simulink model "ModeAdjust"  (R2018b)
settings: Solver=FixedStepDiscrete  StartTime=0.0  StopTime=inf  FixedStep=0.01  RelTol=1e-3
undefined symbols (not defined in the file or in its folder): IfKeSMSbSeatMovBkRclnEnable_Val, IfKeSMSbSeatMovFrwdBkwdEnable_Val, IfKeSMSbSeatMovFtrstEnable_Val, IfKeSMSbSeatMovHdrstFrwdBkwdEnable_Val, IfKeSMSbSeatMovHdUpwdDnwdEnable_Val, IfKeSMSbSeatMovLgrstEnable_Val, IfKeSMSbSeatMovLtwdRtwdEnable_Val, IfVeSMSeStNumConfig, KeSMSbArmscreenMovEnable_Val, KeSMSbSeatMovLgrstExpdEnable_Val, KeSMSuFirstRwStBackPosDelta_Val, KeSMSuFirstRwStBackPosTolr_Val, KeSMSuFirstRwStCushFrntPosDelta_Val, KeSMSuFirstRwStCushFrntPosTolr_Val, KeSMSuFirstRwStCushRePosDelta_Val, KeSMSuFirstRwStCushRePosTolr_Val, KeSMSuFirstRwStFootrestPosDelta_Val, KeSMSuFirstRwStFootrestPosTolr_Val, KeSMSuFirstRwStFwdBkwdPosDelta_Val, KeSMSuFirstRwStFwdBkwdPosTolr_Val, KeSMSuMdMotFinshdTm_Val, KeSMSuMdRetryTm1_Val, KeSMSuModeReqDurgTm_Val, KeSMSuSecRwStArmTochPosDelta_Val, KeSMSuSecRwStArmTochPosTolr_Val, KeSMSuSecRwStBackPosDelta_Val, KeSMSuSecRwStBackPosTolr_Val, KeSMSuSecRwStFtrstUpwdDnwdPosDelta_Val, KeSMSuSecRwStFtrstUpwdDnwdPosTolr_Val, KeSMSuSecRwStFwdBkwdPosDelta_Val, KeSMSuSecRwStFwdBkwdPosTolr_Val, KeSMSuSecRwStHeadrestFwdBkwdPosDelta_Val, KeSMSuSecRwStHeadrestFwdBkwdPosTolr_Val, KeSMSuSecRwStHeadrestUpwdDwnwdPosDelta_Val, KeSMSuSecRwStHeadrestUpwdDwnwdPosTolr_Val, KeSMSuSecRwStLegrestInOutPosDelta_Val, KeSMSuSecRwStLegrestInOutPosTolr_Val, KeSMSuSecRwStLegrestUpwdDwnwdPosDelta_Val, KeSMSuSecRwStLegrestUpwdDwnwdPosTolr_Val, KeSMSuSecRwStLwdRwdPosDelta_Val, KeSMSuSecRwStLwdRwdPosTolr_Val, KeSMSuSecRwStVIPFtrstRefAngle_Val, KeSMSuThirdRwStFwdBkwdPosDelta_Val, KeSMSuThirdRwStFwdBkwdPosTolr_Val, KeSMSuThrdRwCushFoldPosDelta_Val, KeSMSuThrdRwCushFoldPosTolr_Val, KeSMSuThrdRwStBackPosDelta_Val, KeSMSuThrdRwStBackPosTolr_Val, KeSMSw4SLegrstCloseMdSecRwLtStFtrstUpwdDnwdPos_Val, KeSMSw4SLegrstCloseMdSecRwLtStFtrstUpwdDnwdPosMax_Val, KeSMSw4SLegrstCloseMdSecRwLtStFtrstUpwdDnwdPosMin_Val, KeSMSw4SLegrstCloseMdSecRwLtStLgrstOtwdInwdPos_Val, KeSMSw4SLegrstCloseMdSecRwLtStLgrstOtwdInwdPosMax_Val, KeSMSw4SLegrstCloseMdSecRwLtStLgrstOtwdInwdPosMin_Val, KeSMSw4SLegrstCloseMdSecRwLtStLgrstUpwdDnwdPos_Val, KeSMSw4SLegrstCloseMdSecRwLtStLgrstUpwdDnwdPosMax_Val, KeSMSw4SLegrstCloseMdSecRwLtStLgrstUpwdDnwdPosMin_Val, KeSMSw4SLegrstCloseMdSecRwRtStFtrstUpwdDnwdPos_Val, KeSMSw4SLegrstCloseMdSecRwRtStFtrstUpwdDnwdPosMax_Val, KeSMSw4SLegrstCloseMdSecRwRtStFtrstUpwdDnwdPosMin_Val ... (+1138)
libraries: Lib x401
(part 7 of 35)

== system ModeAdjust/ModeAdjustRunnable_sys/ModeAdjust/Default ==
  Bus Creator : BusCreator  Inputs=36  OutDataTypeStr=Bus: isAcsMdFeedBack_Default
  Constant{,43..45} (4 alike) : Constant  Value=0  OutDataTypeStr=uint8
  Constant{1..42} (42 alike) : Constant  Value=0  OutDataTypeStr=boolean
  PA_KeSMSuFirstRwStBackPosDelta_Val : Constant  Value=KeSMSuFirstRwStBackPosDelta_Val
  PA_KeSMSuFirstRwStCushFrntPosDelta_Val : Constant  Value=KeSMSuFirstRwStCushFrntPosDelta_Val
  PA_KeSMSuFirstRwStCushRePosDelta_Val : Constant  Value=KeSMSuFirstRwStCushRePosDelta_Val
  PA_KeSMSuFirstRwStFootrestPosDelta_Val : Constant  Value=KeSMSuFirstRwStFootrestPosDelta_Val
  PA_KeSMSuFirstRwStFwdBkwdPosDelta_Val : Constant  Value=KeSMSuFirstRwStFwdBkwdPosDelta_Val
  PA_KeSMSuMdMotFinshdTm_Val : Constant  Value=KeSMSuMdMotFinshdTm_Val
  PA_KeSMSuSecRwStArmTochPosDelta_Val : Constant  Value=KeSMSuSecRwStArmTochPosDelta_Val
  PA_KeSMSuSecRwStBackPosDelta_Val : Constant  Value=KeSMSuSecRwStBackPosDelta_Val
  PA_KeSMSuSecRwStFwdBkwdPosDelta_Val : Constant  Value=KeSMSuSecRwStFwdBkwdPosDelta_Val
  PA_KeSMSuSecRwStHeadrestFwdBkwdPosDelta_Val : Constant  Value=KeSMSuSecRwStHeadrestFwdBkwdPosDelta_Val
  PA_KeSMSuSecRwStHeadrestUpwdDwnwdPosDelta_Val : Constant  Value=KeSMSuSecRwStHeadrestUpwdDwnwdPosDelta_Val
  PA_KeSMSuSecRwStLegrestInOutPosDelta_Val : Constant  Value=KeSMSuSecRwStLegrestInOutPosDelta_Val
  PA_KeSMSuSecRwStLegrestUpwdDwnwdPosDelta_Val : Constant  Value=KeSMSuSecRwStLegrestUpwdDwnwdPosDelta_Val
  PA_KeSMSuSecRwStLwdRwdPosDelta_Val : Constant  Value=KeSMSuSecRwStLwdRwdPosDelta_Val
  PA_KeSMSuThirdRwStFwdBkwdPosDelta_Val : Constant  Value=KeSMSuThirdRwStFwdBkwdPosDelta_Val
  PA_KeSMSuThrdRwCushFoldPosDelta_Val : Constant  Value=KeSMSuThrdRwCushFoldPosDelta_Val
  PA_KeSMSuThrdRwStBackPosDelta_Val : Constant  Value=KeSMSuThrdRwStBackPosDelta_Val
  Subsystem : Subsystem
  Subsystem1 : Subsystem
  Subsystem2 : Subsystem
  Subsystem3 : Subsystem
  Subsystem4 : Subsystem
  Subsystem5 : Subsystem
  Subsystem6 : Subsystem
  Subsystem7 : Subsystem
  EZE_DrvStTrgtPoss : Outport  VectorParamsAs1DForOutWhenUnconnected=on
  PassStTrgtPoss : Outport  Port=2  VectorParamsAs1DForOutWhenUnconnected=on
  R2Lt_TrgtPoss : Outport  Port=3  VectorParamsAs1DForOutWhenUnconnected=on
  R2Rt_TrgtPoss : Outport  Port=4  VectorParamsAs1DForOutWhenUnconnected=on
  R3Lt_TrgtPoss : Outport  Port=5  VectorParamsAs1DForOutWhenUnconnected=on
  R3Rt_TrgtPoss : Outport  Port=6  VectorParamsAs1DForOutWhenUnconnected=on
  isAcsMdFeedBack_Default : Outport  Port=7
  IfVeSMSbThdRwRtStRclCmdSrv_Val_writeDef : Outport  Port=8
  IfVeSMSbThdRwLtStRclCmdSrv_Val_writeDef : Outport  Port=9
  IfVeSMSbSecRwRtStRclCmdSrv_Val_writeDef : Outport  Port=10
  IfVeSMSuSecRwLtStRclCmdSrv_Val_writeDef : Outport  Port=11
  IfVeSMSbDrvStRclCmdSrv_Val_writeDef : Outport  Port=12
  IfVeSMSuPassStRclCmdSrv_Val_writeDef : Outport  Port=13
  R2Lt_TrgtPoss4s : Outport  Port=14  VectorParamsAs1DForOutWhenUnconnected=on
  R2Rt_TrgtPoss4s : Outport  Port=15  VectorParamsAs1DForOutWhenUnconnected=on
  R2Lt_SpdCtrl : Outport  Port=16  VectorParamsAs1DForOutWhenUnconnected=on
  R2Rt_SpdCtrl : Outport  Port=17  VectorParamsAs1DForOutWhenUnconnected=on
  R3Lt_SpdCtrl : Outport  Port=18  VectorParamsAs1DForOutWhenUnconnected=on
  R3Rt_SpdCtrl : Outport  Port=19  VectorParamsAs1DForOutWhenUnconnected=on
  wires:
  Constant11/1 -> IfVeSMSuSecRwLtStRclCmdSrv_Val_writeDef/1  "IfVeSMSuSecRwLtStRclCmdSrv_Val_write"
  Constant9/1 -> IfVeSMSbDrvStRclCmdSrv_Val_writeDef/1  "IfVeSMSbDrvStRclCmdSrv_Val_write"
  Constant10/1 -> IfVeSMSuPassStRclCmdSrv_Val_writeDef/1  "IfVeSMSuPassStRclCmdSrv_Val_write"
  Constant7/1 -> IfVeSMSbThdRwLtStRclCmdSrv_Val_writeDef/1  "IfVeSMSbThdRwLtStRclCmdSrv_Val_write"
  Constant8/1 -> IfVeSMSbSecRwRtStRclCmdSrv_Val_writeDef/1  "IfVeSMSbSecRwRtStRclCmdSrv_Val_write"
  Constant5/1 -> IfVeSMSbThdRwRtStRclCmdSrv_Val_writeDef/1  "IfVeSMSbThdRwRtStRclCmdSrv_Val_write"
  Constant19/1 -> Bus Creator/15  "isRtLugDoneOK"
  Constant22/1 -> Bus Creator/3  "isAcsMdExtDoneOK"
  Constant23/1 -> Bus Creator/5  "isLfVipDoneOK"
  Constant26/1 -> Bus Creator/8  "isRtVipDoneFailed"
  Constant24/1 -> Bus Creator/6  "isLfVipDoneFailed"
  Constant20/1 -> Bus Creator/1  "isAcsMdEntryDoneOK"
  Constant21/1 -> Bus Creator/2  "isAcsMdEntryDoneFailed"
  Constant2/1 -> Bus Creator/10  "isLfRecoveryDoneFailed"
  Constant17/1 -> Bus Creator/13  "isLfLugDoneOK"
  Constant25/1 -> Bus Creator/7  "isRtVipDoneOK"
  Constant3/1 -> Bus Creator/11  "isRfRecoveryDoneOK"
  Constant18/1 -> Bus Creator/14  "isLfLugDoneFailed"
  Constant6/1 -> Bus Creator/4  "isAcsMdExtDoneFailed"
  Constant1/1 -> Bus Creator/9  "isLfRecoveryDoneOK"
  Bus Creator/1 -> isAcsMdFeedBack_Default/1
  Constant15/1 -> Bus Creator/16  "isRtLugDoneFailed"
  Constant4/1 -> Bus Creator/12  "isRfRecoveryDoneFailed"
  Subsystem/1(DrvStTrgtPoss) -> EZE_DrvStTrgtPoss/1
  Subsystem1/1(PassStTrgtPoss) -> PassStTrgtPoss/1
  Subsystem2/1(R2Lt_TrgtPoss) -> R2Lt_TrgtPoss/1
  Subsystem3/1(R2Rt_TrgtPoss) -> R2Rt_TrgtPoss/1
  Subsystem4/1(R3Lt_TrgtPoss) -> R3Lt_TrgtPoss/1
  Subsystem5/1(R3Rt_TrgtPoss) -> R3Rt_TrgtPoss/1
  PA_KeSMSuFirstRwStFootrestPosDelta_Val/1 -> [KeSMSuFirstRwStFootrestPosDelta_Val]
  PA_KeSMSuSecRwStLegrestInOutPosDelta_Val/1 -> [KeSMSuSecRwStLegrestInOutPosDelta_Val]
  PA_KeSMSuSecRwStLegrestUpwdDwnwdPosDelta_Val/1 -> [KeSMSuSecRwStLegrestUpwdDwnwdPosDelta_Val]
  PA_KeSMSuThrdRwStBackPosDelta_Val/1 -> [KeSMSuThrdRwStBackPosDelta_Val]
  PA_KeSMSuSecRwStFwdBkwdPosDelta_Val/1 -> [KeSMSuSecRwStFwdBkwdPosDelta_Val]
  PA_KeSMSuSecRwStLwdRwdPosDelta_Val/1 -> [KeSMSuSecRwStLwdRwdPosDelta_Val]
  PA_KeSMSuSecRwStArmTochPosDelta_Val/1 -> [KeSMSuSecRwStArmTochPosDelta_Val]
  PA_KeSMSuSecRwStHeadrestUpwdDwnwdPosDelta_Val/1 -> [KeSMSuSecRwStHeadrestUpwdDwnwdPosDelta_Val]
  PA_KeSMSuMdMotFinshdTm_Val/1 -> [KeSMSuMdMotFinshdTm_Val]
  PA_KeSMSuSecRwStHeadrestFwdBkwdPosDelta_Val/1 -> [KeSMSuSecRwStHeadrestFwdBkwdPosDelta_Val]
  PA_KeSMSuSecRwStBackPosDelta_Val/1 -> [KeSMSuSecRwStBackPosDelta_Val]
  PA_KeSMSuFirstRwStFwdBkwdPosDelta_Val/1 -> [KeSMSuFirstRwStFwdBkwdPosDelta_Val]
  PA_KeSMSuFirstRwStCushFrntPosDelta_Val/1 -> [KeSMSuFirstRwStCushFrntPosDelta_Val]
  PA_KeSMSuFirstRwStBackPosDelta_Val/1 -> [KeSMSuFirstRwStBackPosDelta_Val]
  PA_KeSMSuFirstRwStCushRePosDelta_Val/1 -> [KeSMSuFirstRwStCushRePosDelta_Val]
  PA_KeSMSuThirdRwStFwdBkwdPosDelta_Val/1 -> [KeSMSuThirdRwStFwdBkwdPosDelta_Val]
  PA_KeSMSuThrdRwCushFoldPosDelta_Val/1 -> [KeSMSuThrdRwCushFoldPosDelta_Val]
  Constant12/1 -> Bus Creator/17  "isINTMDoneOK"
  Constant13/1 -> Bus Creator/18  "isINTMDoneFailed"
  Constant14/1 -> Bus Creator/19  "isLfFamlyDoneOK"
  Constant16/1 -> Bus Creator/20  "isLfFamlyDoneFailed"
  Constant27/1 -> Bus Creator/21  "isRtFamlyDoneOK"
  Constant28/1 -> Bus Creator/22  "isRtFamlyDoneFailed"
  Constant32/1 -> Bus Creator/26  "isRtLyDoneFailed"
  Constant31/1 -> Bus Creator/25  "isRtLyDoneOK"
  Constant30/1 -> Bus Creator/24  "isLfLyDoneFailed"
  Constant29/1 -> Bus Creator/23  "isLfLyDoneOK"
  Subsystem6/1(R2Lt_TrgtPoss) -> R2Lt_TrgtPoss4s/1
  Subsystem7/1(R2Lt_TrgtPoss) -> R2Rt_TrgtPoss4s/1
  Constant33/1 -> Bus Creator/27  "isLgrstOpenLDoneOK"
  Constant34/1 -> Bus Creator/28  "isLgrstOpenLDoneFailed"
  Constant35/1 -> Bus Creator/29  "isLgrstCloseLDoneOK"
  Constant36/1 -> Bus Creator/30  "isLgrstCloseLDoneFailed"
  Constant37/1 -> Bus Creator/31  "isLgrstOpenRDoneOK"
  Constant38/1 -> Bus Creator/32  "isLgrstOpenRDoneFailed"
  Constant39/1 -> Bus Creator/33  "isLgrstCloseRDoneOK"
  Constant40/1 -> Bus Creator/34  "isLgrstCloseRDoneFailed"
  Constant41/1 -> Bus Creator/35  "isINTMRDoneOK"
  Constant42/1 -> Bus Creator/36  "isINTMRDoneFailed"
  Constant/1 -> R2Lt_SpdCtrl/1
  Constant43/1 -> R2Rt_SpdCtrl/1
  Constant44/1 -> R3Lt_SpdCtrl/1
  Constant45/1 -> R3Rt_SpdCtrl/1

== system ModeAdjust/ModeAdjustRunnable_sys/ModeAdjust/FAMLYL ==
  SecRwLtStsPoss : Inport
  SecRwLtStPossV : Inport  Port=2
  SecRwRtStChldLkRsp_L : Inport  Port=3
  FAMLY_L_En : Inport  Port=4
  ModeStCalib : Inport  Port=5
  ThdRwRtStPoss : Inport  Port=6
  ThdRwRtStPossV : Inport  Port=7
  StConfig : Inport  Port=8
  SecRwRtStPoss : Inport  Port=9
  SecRwRtStPossV : Inport  Port=10
  SecRwRtStChldLkRsp_R : Inport  Port=11
  isLfFamlyArrivedAtTargetPos : Inport  Port=12
  ThdRwLtStPoss : Inport  Port=13
  ThdRwLtStPossV : Inport  Port=14
  Enable : EnablePort  StatesWhenEnabling=reset
  Bus Creator1 : BusCreator  Inputs=2
  Bus Selector : BusSelector  OutputSignals=Calib_Drv,Calib_Pass,Calib_2L,Calib_2R,Calib_3L,Calib_3R
  Bus Selector1 : BusSelector  OutputSignals=DrvStConfig,PassStConfig,SecRwLtStConfig,SecRwRtStConfig,ThdRwLtStConfig,ThdRwRtStConfig
  Chart1 : Stateflow chart  TreatAsAtomicUnit=on
  Chart2 : Stateflow chart  TreatAsAtomicUnit=on
  Logical Operator : Logic  Operator=NOT  AllPortsSameDT=off  OutDataTypeStr=boolean
  Logical Operator12 : Logic  Inputs=4  AllPortsSameDT=off  OutDataTypeStr=boolean
  R2Lt : Subsystem
  R2Rt : Subsystem
  R3Lt : Subsystem
  R3Rt : Subsystem
  VIP_TrigJudg : Lib/VIP_TrigJudg  SystemSampleTime=-1
  R2Lt_TrgtPoss : Outport  VectorParamsAs1DForOutWhenUnconnected=on
  IfVeSMSbSecRwRtStRclCmdSrv_Val_writeFAMLY : Outport  Port=2
  IfVeSMSuSecRwLtStRclCmdSrv_Val_writeFAMLY : Outport  Port=3
  isMdFeedBackNew_FAMLYL : Outport  Port=4
  R3Rt_TrgtPoss : Outport  Port=5  VectorParamsAs1DForOutWhenUnconnected=on
  IfVeSMSbThdRwRtStRclCmdSrv_Val_writeFAMLY : Outport  Port=6
  R2Rt_TrgtPoss : Outport  Port=7  VectorParamsAs1DForOutWhenUnconnected=on
  R3Lt_TrgtPoss : Outport  Port=8  VectorParamsAs1DForOutWhenUnconnected=on
  IfVeSMSbThdRwLtStRclCmdSrv_Val_writeFAMLY : Outport  Port=9
  R2Lt_SpdCtrl : Outport  Port=10  VectorParamsAs1DForOutWhenUnconnected=on
  R2Rt_SpdCtrl : Outport  Port=11  VectorParamsAs1DForOutWhenUnconnected=on
  R3Lt_SpdCtrl : Outport  Port=12  VectorParamsAs1DForOutWhenUnconnected=on
  R3Rt_SpdCtrl : Outport  Port=13  VectorParamsAs1DForOutWhenUnconnected=on
  wires:
  SecRwRtStChldLkRsp_L/1 -> [SecRwRtStChldLkRsp_L], R2Lt/5(SecRwRtStChldLkRsp_L)
  SecRwLtStPossV/1 -> R2Lt/4(SecRwLtStPossV)
  SecRwLtStsPoss/1 -> R2Lt/3(SecRwLtStsPoss)
  R2Lt/2(R2Lt_TrgtPoss) -> R2Lt_TrgtPoss/1
  [FAMLY_TrigL] -> R2Lt/1(Mode_Trig)
  [IfVeSMSbSecRwRtStRclCmdSrv_Val_writeRaw] -> Chart1/2(IfVeSMSbSecRwRtStRclCmdSrv_Val_writeRaw)
  R2Lt/1(R2Lt_Step2_Ini) -> [R2LtST_Step2_ini]
  VIP_TrigJudg/1 -> [FAMLY_TrigL]
  [R3Rt_Step1_ini] -> [R_R3_ini_done]
  [R3Rt_Step1_ini] -> Chart2/5(R_R3_Step1_ini)
  [R3Rt_Step1_done] -> Chart2/6(R_R3_Step1done)
  Chart2/1(R_R3Step1) -> [R_R3Step1]
  Chart2/2(R_R2Step2) -> [R_R2Step2]
  Chart2/3(L_R2Step2) -> [L_R2Step2]
  [R3Rt_Step1_ini] -> [R_R3_ini]
  [L_R2Step2] -> R2Lt/2(Step2En)
  [R2RtST_Step2_ini] -> Chart2/1(R_R2Step2_ini)
  [R2LtST_Step2_ini] -> Chart2/2(L_R2Step2_ini)
  [R2RtST_All_done] -> Chart2/3(R_R2_Step2done)
  [R2LtST_All_done] -> Chart2/4(L_R2_Step2done)
  [R2LtST_Step2_ini] -> [L_R2_ini]
  FAMLY_L_En/1 -> [FAMLY_L_En]
  [IfVeSMSuSecRwLtStRclCmdSrv_Val_writeRaw] -> Chart1/3(IfVeSMSuSecRwLtStRclCmdSrv_Val_writeRaw)
  R2Lt/3(IfVeSMSuSecRwLtStRclCmdSrv_Val_writeRaw) -> [IfVeSMSuSecRwLtStRclCmdSrv_Val_writeRaw]
  [R2LtST_All_done] -> Logical Operator12/2
  [R2RtST_All_done] -> Logical Operator12/1
  [Md_L_MvDoneOK] -> Chart1/4(Md_L_DoneOkRaw)
  [Md_L_MvDoneFailed] -> Chart1/5(Md_L_DoneFailedRaw)
  Chart1/3(Md_L_DoneOk) -> [MD_L_DoneOK]
  Chart1/4(Md_L_DoneFailed) -> [MD_L_DoneFailed]
  Chart1/1(IfVeSMSbSecRwRtStRclCmdSrv_Val_write) -> IfVeSMSbSecRwRtStRclCmdSrv_Val_writeFAMLY/1  "IfVeSMSbSecRwRtStRclCmdSrv_Val_write"
  Chart1/2(IfVeSMSuSecRwLtStRclCmdSrv_Val_write) -> IfVeSMSuSecRwLtStRclCmdSrv_Val_writeFAMLY/1  "IfVeSMSuSecRwLtStRclCmdSrv_Val_write"
  R2Lt/4(R2Lt_All_done) -> [R2LtST_All_done]
  Bus Selector/2 -> [ModeStCalib_Pass]  "<Calib_Pass>"
  Bus Selector/5 -> [ModeStCalib_3L]  "<Calib_3L>"
  Bus Selector/3 -> [ModeStCalib_2L]  "<Calib_2L>"
  Bus Selector/1 -> [ModeStCalib_Drv]  "<Calib_Drv>"
  Bus Selector/6 -> [ModeStCalib_3R]  "<Calib_3R>"
  Bus Selector/4 -> [ModeStCalib_2R]  "<Calib_2R>"
  ModeStCalib/1 -> Bus Selector/1
  [ModeStCalib_2L] -> R2Lt/6(ModeStCalib_2L)
  [FAMLY_L_En] -> VIP_TrigJudg/1
  Bus Creator1/1 -> isMdFeedBackNew_FAMLYL/1
  [MD_L_DoneOK] -> Bus Creator1/1  "isLfFamlyDoneOK"
  [MD_L_DoneFailed] -> Bus Creator1/2  "isLfFamlyDoneFailed"
  R3Rt/4(R3Rt_TrgtPoss) -> R3Rt_TrgtPoss/1
  ThdRwRtStPossV/1 -> R3Rt/4(ThdRwRtStPossV)
  R3Rt/3(IfVeSMSbThdRwRtStRclCmdSrv_Val_writeRaw) -> [IfVeSMSbThdRwRtStRclCmdSrv_Val_writeRaw]
  R3Rt/2(R3Rt__Step1done) -> [R3Rt_Step1_done]
  [FAMLY_TrigL] -> R3Rt/1(Mode_Trig)
  [R_R3Step1] -> R3Rt/2(Step1En)
  ThdRwRtStPoss/1 -> R3Rt/3(ThdRwRtStPoss)
  R3Rt/1(R3Rt_Step1_ini) -> [R3Rt_Step1_ini]
  [ModeStCalib_3R] -> R3Rt/5(ModeStCalib_3R)
  [R3Lt_Step1_done] -> Logical Operator12/3
  [IfVeSMSbThdRwRtStRclCmdSrv_Val_writeRaw] -> Chart1/6(IfVeSMSbThdRwRtStRclCmdSrv_Val_writeRaw)
  Chart1/5(IfVeSMSbThdRwRtStRclCmdSrv_Val_write) -> IfVeSMSbThdRwRtStRclCmdSrv_Val_writeFAMLY/1
  Bus Selector1/6 -> [ThdRwRtStConfig]  "<ThdRwRtStConfig>"
  Bus Selector1/1 -> [DrvStConfig]  "<DrvStConfig>"
  Bus Selector1/3 -> [SecRwLtStConfig]  "<SecRwLtStConfig>"
  Bus Selector1/4 -> [SecRwRtStConfig]  "<SecRwRtStConfig>"
  StConfig/1 -> Bus Selector1/1
  Bus Selector1/2 -> [PassStConfig]  "<PassStConfig>"
  Bus Selector1/5 -> [ThdRwLtStConfig]  "<ThdRwLtStConfig>"
  [SecRwLtStConfig] -> R2Lt/7(StConfig)
  [ThdRwRtStConfig] -> R3Rt/6(StConfig)
  Logical Operator12/1 -> Chart1/1(LeftDone)
  [SecRwRtStChldLkRsp_L] -> R3Rt/7(SecRwRtStChldLkRsp_L)
  [SecRwRtStConfig] -> R2Rt/7(StConfig)
  R2Rt/4(R2Rt_All_done) -> [R2RtST_All_done]
  [R_R2Step2] -> R2Rt/2(Step2En)
  R2Rt/2(R2Rt_TrgtPoss) -> R2Rt_TrgtPoss/1
  SecRwRtStPossV/1 -> R2Rt/4(SecRwRtStPossV)
  SecRwRtStChldLkRsp_R/1 -> [SecRwRtStChldLkRsp_R], R2Lt/8(SecRwRtStChldLkRsp_R)
  [FAMLY_TrigL] -> R2Rt/1(Mode_Trig)
  R2Rt/1(R2RtSt_Step2_ini) -> [R2RtST_Step2_ini]
  R2Rt/3(IfVeSMSbSecRwRtStRclCmdSrv_Val_writeRaw) -> [IfVeSMSbSecRwRtStRclCmdSrv_Val_writeRaw]
  SecRwRtStPoss/1 -> R2Rt/3(SecRwRtStPoss)
  [ModeStCalib_2R] -> R2Rt/6(ModeStCalib_2R)
  [SecRwRtStChldLkRsp_L] -> R2Rt/5(SecRwRtStChldLkRsp_L)
  [SecRwRtStChldLkRsp_R] -> R2Rt/8(SecRwRtStChldLkRsp_R)
  [SecRwRtStChldLkRsp_R] -> R3Rt/8(SecRwRtStChldLkRsp_R)
  Logical Operator/1 -> [Md_L_MvDoneFailed]
  isLfFamlyArrivedAtTargetPos/1 -> [Md_L_MvDoneOK], Logical Operator/1
  [FAMLY_TrigL] -> R3Lt/1(Mode_Trig)
  R3Lt/1(R3Rt_Step1_ini) -> [R3Lt_Step1_ini]
  [L_R3Step1] -> R3Lt/2(Step1En)
  R3Lt/2(R3Lt__Step1done) -> [R3Lt_Step1_done]
  [SecRwRtStChldLkRsp_L] -> R3Lt/7(SecRwRtStChldLkRsp_L)
  R3Lt/3(IfVeSMSbThdRwLtStRclCmdSrv_Val_writeRaw) -> [IfVeSMSbThdRwLtStRclCmdSrv_Val_writeRaw]
  R3Lt/4(R3Lt_TrgtPoss) -> R3Lt_TrgtPoss/1
  [ThdRwLtStConfig] -> R3Lt/6(StConfig)
  ThdRwLtStPoss/1 -> R3Lt/3(ThdRwRtStPoss)
  [ModeStCalib_3L] -> R3Lt/5(ModeStCalib_3R)
  ThdRwLtStPossV/1 -> R3Lt/4(ThdRwRtStPossV)
  [SecRwRtStChldLkRsp_R] -> R3Lt/8(SecRwRtStChldLkRsp_R)
  [R3Rt_Step1_done] -> Logical Operator12/4
  [IfVeSMSbThdRwLtStRclCmdSrv_Val_writeRaw] -> Chart1/7(IfVeSMSbThdRwLtStRclCmdSrv_Val_writeRaw)
  Chart1/6(IfVeSMSbThdRwLtStRclCmdSrv_Val_write) -> IfVeSMSbThdRwLtStRclCmdSrv_Val_writeFAMLY/1
  [R3Lt_Step1_done] -> Chart2/8(L_R3_Step1done)
  [R3Lt_Step1_ini] -> Chart2/7(L_R3_Step1_ini)
  Chart2/4(L_R3Step1) -> [L_R3Step1]
  R2Lt/5(R2Lt_SpdCtrl) -> R2Lt_SpdCtrl/1
  R2Rt/5(R2Rt_SpdCtrl) -> R2Rt_SpdCtrl/1
  R3Lt/5(R3Lt_SpdCtrl) -> R3Lt_SpdCtrl/1
  R3Rt/5(R3Rt_SpdCtrl) -> R3Rt_SpdCtrl/1

== system ModeAdjust/ModeAdjustRunnable_sys/ModeAdjust/FAMLYR ==
  SecRwLtStsPoss : Inport
  SecRwLtStPossV : Inport  Port=2
  SecRwRtStChldLkRsp_L : Inport  Port=3
  FAMLY_L_En : Inport  Port=4
  ModeStCalib : Inport  Port=5
  ThdRwLtStPoss : Inport  Port=6
  ThdRwLtStPossV : Inport  Port=7
  StConfig : Inport  Port=8
  SecRwRtStPoss : Inport  Port=9
  SecRwRtStPossV : Inport  Port=10
  SecRwRtStChldLkRsp_R : Inport  Port=11
  isRtFamlyArrivedAtTargetPos : Inport  Port=12
  ThdRwRtStPoss : Inport  Port=13
  ThdRwRtStPossV : Inport  Port=14
  Enable : EnablePort  StatesWhenEnabling=reset
  Bus Creator1 : BusCreator  Inputs=2
  Bus Selector : BusSelector  OutputSignals=Calib_Drv,Calib_Pass,Calib_2L,Calib_2R,Calib_3L,Calib_3R
  Bus Selector1 : BusSelector  OutputSignals=DrvStConfig,PassStConfig,SecRwLtStConfig,SecRwRtStConfig,ThdRwLtStConfig,ThdRwRtStConfig
  Chart1 : Stateflow chart  TreatAsAtomicUnit=on
  Chart2 : Stateflow chart  TreatAsAtomicUnit=on
  Logical Operator : Logic  Operator=NOT  AllPortsSameDT=off  OutDataTypeStr=boolean
  Logical Operator12 : Logic  Inputs=4  AllPortsSameDT=off  OutDataTypeStr=boolean
  R2Lt1 : Subsystem
  R2Rt1 : Subsystem
  R3Lt : Subsystem
  R3Rt : Subsystem
  VIP_TrigJudg : Lib/VIP_TrigJudg  SystemSampleTime=-1
  R2Lt_TrgtPoss : Outport  VectorParamsAs1DForOutWhenUnconnected=on
  IfVeSMSbSecRwRtStRclCmdSrv_Val_writeFAMLY : Outport  Port=2
  IfVeSMSuSecRwLtStRclCmdSrv_Val_writeFAMLY : Outport  Port=3
  isMdFeedBackNew_FAMLYR : Outport  Port=4
  R3Lt_TrgtPoss : Outport  Port=5  VectorParamsAs1DForOutWhenUnconnected=on
  IfVeSMSbThdRwLtStRclCmdSrv_Val_writeFAMLY : Outport  Port=6
  R2Rt_TrgtPoss : Outport  Port=7  VectorParamsAs1DForOutWhenUnconnected=on
  R3Rt_TrgtPoss : Outport  Port=8  VectorParamsAs1DForOutWhenUnconnected=on
  IfVeSMSbThdRwRtStRclCmdSrv_Val_writeFAMLY : Outport  Port=9
  R2Lt_SpdCtrl : Outport  Port=10  VectorParamsAs1DForOutWhenUnconnected=on
  R2Rt_SpdCtrl : Outport  Port=11  VectorParamsAs1DForOutWhenUnconnected=on
  R3Lt_SpdCtrl : Outport  Port=12  VectorParamsAs1DForOutWhenUnconnected=on
  R3Rt_SpdCtrl : Outport  Port=13  VectorParamsAs1DForOutWhenUnconnected=on
  wires:
  SecRwRtStChldLkRsp_L/1 -> R2Lt1/5(SecRwRtStChldLkRsp_L), [SecRwRtStChldLkRsp_L]
  SecRwLtStPossV/1 -> R2Lt1/4(SecRwLtStPossV)
  SecRwLtStsPoss/1 -> R2Lt1/3(SecRwLtStsPoss)
  R2Lt1/2(R2Lt_TrgtPoss) -> R2Lt_TrgtPoss/1
  [FAMLY_TrigL] -> R2Lt1/1(Mode_Trig)
  [IfVeSMSbSecRwRtStRclCmdSrv_Val_writeRaw] -> Chart1/2(IfVeSMSbSecRwRtStRclCmdSrv_Val_writeRaw)
  R2Lt1/1(R2Lt_Step2_Ini) -> [R2LtST_Step2_ini]
  VIP_TrigJudg/1 -> [FAMLY_TrigL]
  [R3Rt_Step1_ini] -> [R_R3_ini_done]
  [R3Rt_Step1_ini] -> Chart2/5(R_R3_Step1_ini)
  [R3Rt_Step1_done] -> Chart2/6(R_R3_Step1done)
  Chart2/1(R_R3Step1) -> [R_R3Step1]
  Chart2/2(R_R2Step2) -> [R_R2Step2]
  Chart2/3(L_R2Step2) -> [L_R2Step2]
  [R3Rt_Step1_ini] -> [R_R3_ini]
  [L_R2Step2] -> R2Lt1/2(Step2En)
  [R2RtST_Step2_ini] -> Chart2/1(R_R2Step2_ini)
  [R2LtST_Step2_ini] -> Chart2/2(L_R2Step2_ini)
  [R2RtST_All_done] -> Chart2/3(R_R2_Step2done)
  [R2LtST_All_done] -> Chart2/4(L_R2_Step2done)
  [R2LtST_Step2_ini] -> [L_R2_ini]
  FAMLY_L_En/1 -> [FAMLY_L_En]
  [IfVeSMSuSecRwLtStRclCmdSrv_Val_writeRaw] -> Chart1/3(IfVeSMSuSecRwLtStRclCmdSrv_Val_writeRaw)
  R2Lt1/3(IfVeSMSuSecRwLtStRclCmdSrv_Val_writeRaw) -> [IfVeSMSuSecRwLtStRclCmdSrv_Val_writeRaw]
  [R2LtST_All_done] -> Logical Operator12/2
  [R2RtST_All_done] -> Logical Operator12/1
  [Md_L_MvDoneOK] -> Chart1/4(Md_L_DoneOkRaw)
  [Md_L_MvDoneFailed] -> Chart1/5(Md_L_DoneFailedRaw)
  Chart1/3(Md_L_DoneOk) -> [MD_L_DoneOK]
  Chart1/4(Md_L_DoneFailed) -> [MD_L_DoneFailed]
  Chart1/1(IfVeSMSbSecRwRtStRclCmdSrv_Val_write) -> IfVeSMSbSecRwRtStRclCmdSrv_Val_writeFAMLY/1  "IfVeSMSbSecRwRtStRclCmdSrv_Val_write"
  Chart1/2(IfVeSMSuSecRwLtStRclCmdSrv_Val_write) -> IfVeSMSuSecRwLtStRclCmdSrv_Val_writeFAMLY/1  "IfVeSMSuSecRwLtStRclCmdSrv_Val_write"
  R2Lt1/4(R2Lt_All_done) -> [R2LtST_All_done]
  Bus Selector/2 -> [ModeStCalib_Pass]  "<Calib_Pass>"
  Bus Selector/5 -> [ModeStCalib_3L]  "<Calib_3L>"
  Bus Selector/3 -> [ModeStCalib_2L]  "<Calib_2L>"
  Bus Selector/1 -> [ModeStCalib_Drv]  "<Calib_Drv>"
  Bus Selector/6 -> [ModeStCalib_3R]  "<Calib_3R>"
  Bus Selector/4 -> [ModeStCalib_2R]  "<Calib_2R>"
  ModeStCalib/1 -> Bus Selector/1
  [ModeStCalib_2L] -> R2Lt1/6(ModeStCalib_2L)
  [FAMLY_L_En] -> VIP_TrigJudg/1
  Bus Creator1/1 -> isMdFeedBackNew_FAMLYR/1
  [MD_L_DoneOK] -> Bus Creator1/1  "isRtFamlyDoneOK"
  [MD_L_DoneFailed] -> Bus Creator1/2  "isRtFamlyDoneFailed"
  R3Lt/4(R3Lt_TrgtPoss) -> R3Lt_TrgtPoss/1
  ThdRwLtStPossV/1 -> R3Lt/4(ThdRwRtStPossV)
  R3Lt/3(IfVeSMSbThdRwLtStRclCmdSrv_Val_writeRaw) -> [IfVeSMSbThdRwLtStRclCmdSrv_Val_writeRaw]
  R3Lt/2(R3Lt__Step1done) -> [R3Lt_Step1_done]
  [FAMLY_TrigL] -> R3Lt/1(Mode_Trig)
  [L_R3Step1] -> R3Lt/2(Step1En)
  ThdRwLtStPoss/1 -> R3Lt/3(ThdRwRtStPoss)
  R3Lt/1(R3Rt_Step1_ini) -> [R3Lt_Step1_ini]
  [ModeStCalib_3L] -> R3Lt/5(ModeStCalib_3R)
  [IfVeSMSbThdRwRtStRclCmdSrv_Val_writeRaw] -> Chart1/6(IfVeSMSbThdRwRtStRclCmdSrv_Val_writeRaw)
  Bus Selector1/6 -> [ThdRwRtStConfig]  "<ThdRwRtStConfig>"
  Bus Selector1/1 -> [DrvStConfig]  "<DrvStConfig>"
  Bus Selector1/3 -> [SecRwLtStConfig]  "<SecRwLtStConfig>"
  Bus Selector1/4 -> [SecRwRtStConfig]  "<SecRwRtStConfig>"
  StConfig/1 -> Bus Selector1/1
  Bus Selector1/2 -> [PassStConfig]  "<PassStConfig>"
  Bus Selector1/5 -> [ThdRwLtStConfig]  "<ThdRwLtStConfig>"
  [SecRwLtStConfig] -> R2Lt1/7(StConfig)
  [ThdRwLtStConfig] -> R3Lt/6(StConfig)
  Logical Operator12/1 -> Chart1/1(LeftDone)
  [SecRwRtStChldLkRsp_L] -> R3Lt/7(SecRwRtStChldLkRsp_L)
  [SecRwRtStConfig] -> R2Rt1/7(StConfig)
  R2Rt1/4(R2Rt_All_done) -> [R2RtST_All_done]
  [R_R2Step2] -> R2Rt1/2(Step2En)
  R2Rt1/2(R2Rt_TrgtPoss) -> R2Rt_TrgtPoss/1
  SecRwRtStPossV/1 -> R2Rt1/4(SecRwRtStPossV)
  SecRwRtStChldLkRsp_R/1 -> R2Lt1/8(SecRwRtStChldLkRsp_R), [SecRwRtStChldLkRsp_R]
  [FAMLY_TrigL] -> R2Rt1/1(Mode_Trig)
  R2Rt1/1(R2RtSt_Step2_ini) -> [R2RtST_Step2_ini]
  R2Rt1/3(IfVeSMSbSecRwRtStRclCmdSrv_Val_writeRaw) -> [IfVeSMSbSecRwRtStRclCmdSrv_Val_writeRaw]
  SecRwRtStPoss/1 -> R2Rt1/3(SecRwRtStPoss)
  [ModeStCalib_2R] -> R2Rt1/6(ModeStCalib_2R)
  [SecRwRtStChldLkRsp_L] -> R2Rt1/5(SecRwRtStChldLkRsp_L)
  [SecRwRtStChldLkRsp_R] -> R2Rt1/8(SecRwRtStChldLkRsp_R)
  [SecRwRtStChldLkRsp_R] -> R3Lt/8(SecRwRtStChldLkRsp_R)
  Logical Operator/1 -> [Md_L_MvDoneFailed]
  isRtFamlyArrivedAtTargetPos/1 -> [Md_L_MvDoneOK], Logical Operator/1
  [SecRwRtStChldLkRsp_L] -> R3Rt/7(SecRwRtStChldLkRsp_L)
  [ThdRwRtStConfig] -> R3Rt/6(StConfig)
  R3Rt/1(R3Rt_Step1_ini) -> [R3Rt_Step1_ini]
  [SecRwRtStChldLkRsp_R] -> R3Rt/8(SecRwRtStChldLkRsp_R)
  [ModeStCalib_3R] -> R3Rt/5(ModeStCalib_3R)
  R3Rt/4(R3Rt_TrgtPoss) -> R3Rt_TrgtPoss/1
  R3Rt/3(IfVeSMSbThdRwRtStRclCmdSrv_Val_writeRaw) -> [IfVeSMSbThdRwRtStRclCmdSrv_Val_writeRaw]
  ThdRwRtStPoss/1 -> R3Rt/3(ThdRwRtStPoss)
  [FAMLY_TrigL] -> R3Rt/1(Mode_Trig)
  [R_R3Step1] -> R3Rt/2(Step1En)
  ThdRwRtStPossV/1 -> R3Rt/4(ThdRwRtStPossV)
  R3Rt/2(R3Rt__Step1done) -> [R3Rt_Step1_done]
  [R3Lt_Step1_done] -> Logical Operator12/3
  [R3Rt_Step1_done] -> Logical Operator12/4
  Chart1/5(IfVeSMSbThdRwRtStRclCmdSrv_Val_write) -> IfVeSMSbThdRwRtStRclCmdSrv_Val_writeFAMLY/1
  [IfVeSMSbThdRwLtStRclCmdSrv_Val_writeRaw] -> Chart1/7(IfVeSMSbThdRwLtStRclCmdSrv_Val_writeRaw)
  Chart1/6(IfVeSMSbThdRwLtStRclCmdSrv_Val_write) -> IfVeSMSbThdRwLtStRclCmdSrv_Val_writeFAMLY/1
  [R3Lt_Step1_ini] -> Chart2/7(L_R3_Step1_ini)
  [R3Lt_Step1_done] -> Chart2/8(L_R3_Step1done)
  Chart2/4(L_R3Step1) -> [L_R3Step1]
  R2Rt1/5(R2Rt_SpdCtrl) -> R2Rt_SpdCtrl/1
  R2Lt1/5(R2Lt_SpdCtrl) -> R2Lt_SpdCtrl/1
  R3Rt/5(R3Rt_SpdCtrl) -> R3Rt_SpdCtrl/1
  R3Lt/5(R3Lt_SpdCtrl) -> R3Lt_SpdCtrl/1

== system ModeAdjust/ModeAdjustRunnable_sys/ModeAdjust/INTML ==
  note: Change Request 179276
      | 原亲密模式只有二排座椅的左右运动，现在需要做增加前后运动，使二排两侧座椅前后一致；
  INTM_En : Inport
  SecRwLtStsPoss : Inport  Port=2
  SecRwLtStPossV : Inport  Port=3
  SecRwRtStPoss : Inport  Port=4
  SecRwRtStPossV : Inport  Port=5
  SecRwRtStChldLkRsp_L : Inport  Port=6
  SecRwRtStChldLkRsp_R : Inport  Port=7
  ModeStCalib : Inport  Port=8
  StConfig : Inport  Port=9
  isINTMArrivedAtTargetPos : Inport  Port=10
  Enable : EnablePort  StatesWhenEnabling=reset
  Bus Creator1 : BusCreator  Inputs=2
  Bus Selector : BusSelector  OutputSignals=Calib_Drv,Calib_Pass,Calib_2L,Calib_2R,Calib_3L,Calib_3R
  Bus Selector1 : BusSelector  OutputSignals=DrvStConfig,PassStConfig,SecRwLtStConfig,SecRwRtStConfig,ThdRwLtStConfig,ThdRwRtStConfig
  Chart : Stateflow chart  TreatAsAtomicUnit=on
  Chart1 : Stateflow chart  TreatAsAtomicUnit=on
  Delay : Delay  DelayLength=1
  EZE_TrigJudg : Lib/EZE_TrigJudg  SystemSampleTime=-1
  Logical Operator : Logic  Operator=NOT  AllPortsSameDT=off  OutDataTypeStr=boolean
  Logical Operator3 : Logic  AllPortsSameDT=off  OutDataTypeStr=boolean
  Logical Operator6 : Logic  AllPortsSameDT=off  OutDataTypeStr=boolean
  Logical Operator7 : Logic  Operator=OR  AllPortsSameDT=off  OutDataTypeStr=boolean
  R2Lt : Subsystem
  R2Rt : Subsystem
  R2Lt_TrgtPoss : Outport  VectorParamsAs1DForOutWhenUnconnected=on
  R2Rt_TrgtPoss : Outport  Port=2  VectorParamsAs1DForOutWhenUnconnected=on
  IfVeSMSbSecRwRtStRclCmdSrv_Val_writeINTM : Outport  Port=3
  IfVeSMSuSecRwLtStRclCmdSrv_Val_writeINTM : Outport  Port=4
  isAcsMdFeedBackNew_INTM : Outport  Port=5
  R2Lt_SpdCtrl : Outport  Port=6  VectorParamsAs1DForOutWhenUnconnected=on
  wires:
  SecRwRtStChldLkRsp_L/1 -> R2Lt/5(SecRwRtStChldLkRsp_L), [SecRwRtStChldLkRsp_L]
  SecRwRtStPossV/1 -> R2Rt/4(SecRwRtStPossV)
  SecRwRtStPoss/1 -> [SecRwRtStPoss], R2Rt/3(SecRwRtStPoss)
  SecRwLtStPossV/1 -> R2Lt/4(SecRwLtStPossV)
  SecRwLtStsPoss/1 -> R2Lt/3(SecRwLtStsPoss)
  R2Rt/3(R2Rt_TrgtPoss) -> R2Rt_TrgtPoss/1
  R2Lt/3(R2Lt_TrgtPoss) -> R2Lt_TrgtPoss/1
  [INTM_Trig] -> R2Lt/1(Mode_Trig)
  [INTM_Trig] -> R2Rt/1(Mode_Trig)
  Chart1/3(isINTMDoneOk) -> [isINTMDoneOk_OUT]
  Chart1/4(isINTMDoneFailed) -> [isINTMDoneFailed_OUT]
  [R2RtST_Step1_done] -> Logical Operator6/2
  [R2LtST_Step1_done] -> Logical Operator6/1
  R2Rt/2(R2Rt_Step2_done) -> [R2RtST_Step1_done]
  R2Lt/2(R2Lt_Step2_done) -> [R2LtST_Step1_done]
  R2Rt/1(R2RtSt_Step2_ini) -> [R2RtST_Step1_ini]
  R2Lt/1(R2Lt_Ini) -> [R2LtST_Step1_ini]
  Delay/1 -> Logical Operator7/2
  [Stg1_ini_done] -> Logical Operator7/1
  Logical Operator7/1 -> [Stage1MvDone]
  Logical Operator6/1 -> Delay/1
  Chart/1(R_R2_en) -> [R2St_RtEn_Step1]
  Chart/2(L_R2_en) -> [R2ST_LtEn_Step1]
  Logical Operator3/1 -> [Stg1_ini_done]
  EZE_TrigJudg/1 -> [INTM_Trig]
  INTM_En/1 -> EZE_TrigJudg/1
  [R2ST_LtEn_Step1] -> R2Lt/2(Step1En)
  [R2St_RtEn_Step1] -> R2Rt/2(Step1En)
  [isINTMDoneOk] -> Chart1/5(isINTMDoneOkRaw)
  [isINTMDoneFailed] -> Chart1/4(isINTMDoneFailedRaw)
  [IfVeSMSuSecRwLtStRclCmdSrv_Val_writeRaw] -> Chart1/3(IfVeSMSuSecRwLtStRclCmdSrv_Val_writeRaw)
  [IfVeSMSbSecRwRtStRclCmdSrv_Val_writeRaw] -> Chart1/2(IfVeSMSbSecRwRtStRclCmdSrv_Val_writeRaw)
  R2Rt/4(IfVeSMSbSecRwRtStRclCmdSrv_Val_writeRaw) -> [IfVeSMSbSecRwRtStRclCmdSrv_Val_writeRaw]
  R2Lt/4(IfVeSMSuSecRwLtStRclCmdSrv_Val_writeRaw) -> [IfVeSMSuSecRwLtStRclCmdSrv_Val_writeRaw]
  Chart1/1(IfVeSMSbSecRwRtStRclCmdSrv_Val_write) -> IfVeSMSbSecRwRtStRclCmdSrv_Val_writeINTM/1  "IfVeSMSbSecRwRtStRclCmdSrv_Val_write"
  Chart1/2(IfVeSMSuSecRwLtStRclCmdSrv_Val_write) -> IfVeSMSuSecRwLtStRclCmdSrv_Val_writeINTM/1  "IfVeSMSuSecRwLtStRclCmdSrv_Val_write"
  [Stage1MvDone] -> [StageDone]
  [StageDone] -> Chart1/1(StepAlldone)
  Bus Selector/2 -> [ModeStCalib_Pass]  "<Calib_Pass>"
  Bus Selector/5 -> [ModeStCalib_3L]  "<Calib_3L>"
  Bus Selector/3 -> [ModeStCalib_2L]  "<Calib_2L>"
  Bus Selector/1 -> [ModeStCalib_Drv]  "<Calib_Drv>"
  Bus Selector/6 -> [ModeStCalib_3R]  "<Calib_3R>"
  Bus Selector/4 -> [ModeStCalib_2R]  "<Calib_2R>"
  ModeStCalib/1 -> Bus Selector/1
  [ModeStCalib_2L] -> R2Lt/6(ModeStCalib_2L)
  [ModeStCalib_2R] -> R2Rt/6(ModeStCalib_2R)
  [isINTMDoneOk_OUT] -> Bus Creator1/1  "isINTMDoneOK"
  [isINTMDoneFailed_OUT] -> Bus Creator1/2  "isINTMDoneFailed"
  Bus Creator1/1 -> isAcsMdFeedBackNew_INTM/1
  Bus Selector1/6 -> [ThdRwRtStConfig]  "<ThdRwRtStConfig>"
  Bus Selector1/1 -> [DrvStConfig]  "<DrvStConfig>"
  Bus Selector1/3 -> [SecRwLtStConfig]  "<SecRwLtStConfig>"
  Bus Selector1/4 -> [SecRwRtStConfig]  "<SecRwRtStConfig>"
  StConfig/1 -> Bus Selector1/1
  Bus Selector1/2 -> [PassStConfig]  "<PassStConfig>"
  Bus Selector1/5 -> [ThdRwLtStConfig]  "<ThdRwLtStConfig>"
  [SecRwLtStConfig] -> R2Lt/7(StConfig)
  [SecRwRtStConfig] -> R2Rt/7(StConfig)
  [R2RtST_Step1_ini] -> Logical Operator3/2
  [R2LtST_Step1_ini] -> Logical Operator3/1
  [R2LtST_Step1_ini] -> Chart/1(L_R2_ini)
  [R2LtST_Step1_done] -> Chart/2(L_R2_done)
  [R2RtST_Step1_ini] -> Chart/3(R_R2_ini)
  [R2RtST_Step1_done] -> Chart/4(R_R2_done)
  SecRwRtStChldLkRsp_R/1 -> R2Lt/8(SecRwRtStChldLkRsp_R), [SecRwRtStChldLkRsp_R]
  [SecRwRtStChldLkRsp_R] -> R2Rt/8(SecRwRtStChldLkRsp_R)
  [SecRwRtStChldLkRsp_L] -> R2Rt/5(SecRwRtStChldLkRsp_L)
  Logical Operator/1 -> [isINTMDoneFailed]
  isINTMArrivedAtTargetPos/1 -> [isINTMDoneOk], Logical Operator/1
  [SecRwRtStPoss] -> R2Lt/9(SecRwRtStPoss)
  R2Lt/5(R2Lt_SpdCtrl) -> R2Lt_SpdCtrl/1

== system ModeAdjust/ModeAdjustRunnable_sys/ModeAdjust/INTMR ==
  note: Change Request 179276
      | 原亲密模式只有二排座椅的左右运动，现在需要做增加前后运动，使二排两侧座椅前后一致；
  INTM_En : Inport
  SecRwLtStsPoss : Inport  Port=2
  SecRwLtStPossV : Inport  Port=3
  SecRwRtStPoss : Inport  Port=4
  SecRwRtStPossV : Inport  Port=5
  SecRwRtStChldLkRsp_L : Inport  Port=6
  SecRwRtStChldLkRsp_R : Inport  Port=7
  ModeStCalib : Inport  Port=8
  StConfig : Inport  Port=9
  isINTMArrivedAtTargetPos : Inport  Port=10
  Enable : EnablePort  StatesWhenEnabling=reset
  Bus Creator1 : BusCreator  Inputs=2
  Bus Selector : BusSelector  OutputSignals=Calib_Drv,Calib_Pass,Calib_2L,Calib_2R,Calib_3L,Calib_3R
  Bus Selector1 : BusSelector  OutputSignals=DrvStConfig,PassStConfig,SecRwLtStConfig,SecRwRtStConfig,ThdRwLtStConfig,ThdRwRtStConfig
  Chart : Stateflow chart  TreatAsAtomicUnit=on
  Chart1 : Stateflow chart  TreatAsAtomicUnit=on
  Delay : Delay  DelayLength=1
  EZE_TrigJudg : Lib/EZE_TrigJudg  SystemSampleTime=-1
  Logical Operator : Logic  Operator=NOT  AllPortsSameDT=off  OutDataTypeStr=boolean
  Logical Operator3 : Logic  AllPortsSameDT=off  OutDataTypeStr=boolean
  Logical Operator6 : Logic  AllPortsSameDT=off  OutDataTypeStr=boolean
  Logical Operator7 : Logic  Operator=OR  AllPortsSameDT=off  OutDataTypeStr=boolean
  R2Lt : Subsystem
  R2Rt : Subsystem
  R2Lt_TrgtPoss : Outport  VectorParamsAs1DForOutWhenUnconnected=on
  R2Rt_TrgtPoss : Outport  Port=2  VectorParamsAs1DForOutWhenUnconnected=on
  IfVeSMSbSecRwRtStRclCmdSrv_Val_writeINTM : Outport  Port=3
  IfVeSMSuSecRwLtStRclCmdSrv_Val_writeINTM : Outport  Port=4
  isAcsMdFeedBackNew_INTM : Outport  Port=5
  R2Rt_SpdCtrl : Outport  Port=6  VectorParamsAs1DForOutWhenUnconnected=on
  wires:
  isINTMArrivedAtTargetPos/1 -> Logical Operator/1, [isINTMDoneOk]
  Logical Operator/1 -> [isINTMDoneFailed]
  [SecRwRtStChldLkRsp_L] -> R2Rt/5(SecRwRtStChldLkRsp_L)
  [SecRwRtStChldLkRsp_R] -> R2Rt/8(SecRwRtStChldLkRsp_R)
  SecRwRtStChldLkRsp_R/1 -> [SecRwRtStChldLkRsp_R], R2Lt/8(SecRwRtStChldLkRsp_R)
  [R2RtST_Step1_done] -> Chart/4(R_R2_done)
  [R2RtST_Step1_ini] -> Chart/3(R_R2_ini)
  [R2LtST_Step1_done] -> Chart/2(L_R2_done)
  [R2LtST_Step1_ini] -> Chart/1(L_R2_ini)
  [R2LtST_Step1_ini] -> Logical Operator3/1
  [R2RtST_Step1_ini] -> Logical Operator3/2
  [SecRwRtStConfig] -> R2Rt/7(StConfig)
  [SecRwLtStConfig] -> R2Lt/7(StConfig)
  Bus Selector1/5 -> [ThdRwLtStConfig]  "<ThdRwLtStConfig>"
  Bus Selector1/2 -> [PassStConfig]  "<PassStConfig>"
  StConfig/1 -> Bus Selector1/1
  Bus Selector1/4 -> [SecRwRtStConfig]  "<SecRwRtStConfig>"
  Bus Selector1/3 -> [SecRwLtStConfig]  "<SecRwLtStConfig>"
  Bus Selector1/1 -> [DrvStConfig]  "<DrvStConfig>"
  Bus Selector1/6 -> [ThdRwRtStConfig]  "<ThdRwRtStConfig>"
  Bus Creator1/1 -> isAcsMdFeedBackNew_INTM/1
  [isINTMDoneFailed_OUT] -> Bus Creator1/2  "isINTMRDoneFailed"
  [isINTMDoneOk_OUT] -> Bus Creator1/1  "isINTMRDoneOK"
  [ModeStCalib_2R] -> R2Rt/6(ModeStCalib_2R)
  [ModeStCalib_2L] -> R2Lt/6(ModeStCalib_2L)
  ModeStCalib/1 -> Bus Selector/1
  Bus Selector/4 -> [ModeStCalib_2R]  "<Calib_2R>"
  Bus Selector/6 -> [ModeStCalib_3R]  "<Calib_3R>"
  Bus Selector/1 -> [ModeStCalib_Drv]  "<Calib_Drv>"
  Bus Selector/3 -> [ModeStCalib_2L]  "<Calib_2L>"
  Bus Selector/5 -> [ModeStCalib_3L]  "<Calib_3L>"
  Bus Selector/2 -> [ModeStCalib_Pass]  "<Calib_Pass>"
  [StageDone] -> Chart1/1(StepAlldone)
  [Stage1MvDone] -> [StageDone]
  Chart1/2(IfVeSMSuSecRwLtStRclCmdSrv_Val_write) -> IfVeSMSuSecRwLtStRclCmdSrv_Val_writeINTM/1  "IfVeSMSuSecRwLtStRclCmdSrv_Val_write"
  Chart1/1(IfVeSMSbSecRwRtStRclCmdSrv_Val_write) -> IfVeSMSbSecRwRtStRclCmdSrv_Val_writeINTM/1  "IfVeSMSbSecRwRtStRclCmdSrv_Val_write"
  R2Lt/4(IfVeSMSuSecRwLtStRclCmdSrv_Val_writeRaw) -> [IfVeSMSuSecRwLtStRclCmdSrv_Val_writeRaw]
  R2Rt/4(IfVeSMSbSecRwRtStRclCmdSrv_Val_writeRaw) -> [IfVeSMSbSecRwRtStRclCmdSrv_Val_writeRaw]
  [IfVeSMSbSecRwRtStRclCmdSrv_Val_writeRaw] -> Chart1/2(IfVeSMSbSecRwRtStRclCmdSrv_Val_writeRaw)
  [IfVeSMSuSecRwLtStRclCmdSrv_Val_writeRaw] -> Chart1/3(IfVeSMSuSecRwLtStRclCmdSrv_Val_writeRaw)
  [isINTMDoneFailed] -> Chart1/4(isINTMDoneFailedRaw)
  [isINTMDoneOk] -> Chart1/5(isINTMDoneOkRaw)
  [R2St_RtEn_Step1] -> R2Rt/2(Step1En)
  [R2ST_LtEn_Step1] -> R2Lt/2(Step1En)
  INTM_En/1 -> EZE_TrigJudg/1
  EZE_TrigJudg/1 -> [INTM_Trig]
  Logical Operator3/1 -> [Stg1_ini_done]
  Chart/2(L_R2_en) -> [R2ST_LtEn_Step1]
  Chart/1(R_R2_en) -> [R2St_RtEn_Step1]
  Logical Operator6/1 -> Delay/1
  Logical Operator7/1 -> [Stage1MvDone]
  [Stg1_ini_done] -> Logical Operator7/1
  Delay/1 -> Logical Operator7/2
  R2Lt/1(R2Lt_Ini) -> [R2LtST_Step1_ini]
  R2Rt/1(R2RtSt_Step2_ini) -> [R2RtST_Step1_ini]
  R2Lt/2(R2Lt_Step2_done) -> [R2LtST_Step1_done]
  R2Rt/2(R2Rt_Step2_done) -> [R2RtST_Step1_done]
  [R2LtST_Step1_done] -> Logical Operator6/1
  [R2RtST_Step1_done] -> Logical Operator6/2
  Chart1/4(isINTMDoneFailed) -> [isINTMDoneFailed_OUT]
  Chart1/3(isINTMDoneOk) -> [isINTMDoneOk_OUT]
  [INTM_Trig] -> R2Rt/1(Mode_Trig)
  [INTM_Trig] -> R2Lt/1(Mode_Trig)
  R2Lt/3(R2Lt_TrgtPoss) -> R2Lt_TrgtPoss/1
  R2Rt/3(R2Rt_TrgtPoss) -> R2Rt_TrgtPoss/1
  SecRwLtStPossV/1 -> R2Lt/4(SecRwLtStPossV)
  SecRwRtStPoss/1 -> R2Rt/3(SecRwRtStPoss)
  SecRwRtStPossV/1 -> R2Rt/4(SecRwRtStPossV)
  SecRwRtStChldLkRsp_L/1 -> R2Lt/5(SecRwRtStChldLkRsp_L), [SecRwRtStChldLkRsp_L]
  SecRwLtStsPoss/1 -> [SecRwLtStsPoss], R2Lt/3(SecRwLtStsPoss)
  [SecRwLtStsPoss] -> R2Rt/9(SecRwLtStsPoss)
  R2Rt/5(R2Rt_SpdCtrl) -> R2Rt_SpdCtrl/1

== system ModeAdjust/ModeAdjustRunnable_sys/ModeAdjust/LgrstCloseL ==
  note: Change Request 179276
      | 复位模式头枕上下移动到第一步，第一步直接控制靠背、头枕上下、腿托系统同时运动，
      | 当腿托系统运动完成后进行头枕前后运动
  SecRwLtStsPoss : Inport
  SecRwLtStPossV : Inport  Port=2
  Recovery_Mod_Left : Inport  Port=3
  ModeStCalib : Inport  Port=4
  StConfig : Inport  Port=5
  SecRwLtStsPoss4s : Inport  Port=6
  SecRwLtStPossV4s : Inport  Port=7
  StConfig4s : Inport  Port=8
  isLfRecoveryArrivedAtTargetPos : Inport  Port=9
  Enable : EnablePort  StatesWhenEnabling=reset
  Bus Creator1 : BusCreator  Inputs=2
  Bus Selector : BusSelector  OutputSignals=Calib_Drv,Calib_Pass,Calib_2L,Calib_2R,Calib_3L,Calib_3R,Calib_2L4s,Calib_2R4s
  Bus Selector1 : BusSelector  OutputSignals=DrvStConfig,PassStConfig,SecRwLtStConfig,SecRwRtStConfig,ThdRwLtStConfig,ThdRwRtStConfig
  Bus Selector2 : BusSelector  OutputSignals=SecRwLtStConfig,SecRwRtStConfig
  Bus Selector3 : BusSelector  OutputSignals=IfVeSMSuSecRwLtStBkReclnUpwdDnwdPos_Val_read,IfVeSMSuSecRwLtStFrwdBkwdPos_Val_read,IfVeSMSuSecRwLtStHPassStUpwdDnwdPos_Val_read,IfVeSMSuSecRwLtStLgrstUpwdDnwdPos_Val_read,IfVeSMSuSecRwLtStLtwdRtwdPos_Val_read,IfVeSMSuSecRwLtStArmScrnPos_Val_read
  Bus Selector4 : BusSelector  OutputSignals=IfVeSMSuSecRwLtStBkReclnUpwdDnwdPosV_Val_read,IfVeSMSuSecRwLtStFrwdBkwdPosV_Val_read,IfVeSMSuSecRwLtStHPassStUpwdDnwdPosV_Val_read,IfVeSMSuSecRwLtStLgrstUpwdDnwdPosV_Val_read,IfVeSMSuSecRwLtStLtwdRtwdPosV_Val_read,IfVeSMSuSecRwLtStArmScrnPosV_Val_read
  Bus Selector5 : BusSelector  OutputSignals=IfVeSMSuSecRwLtStLgrstOtwdInwdPos_Val_read,IfVeSMSuRrLtStFtUpwdDnwdPos_Val_read,IfVeSMSuSecRwLtStHdrstFrwdBkwdPos_Val_read
  Bus Selector6 : BusSelector  OutputSignals=IfVeSMSuSecRwLtStLgrstOtwdInwdPosV_Val_read,IfVeSMSuRrLtStFtUpwdDnwdPosV_Val_read
  Chart : Stateflow chart  TreatAsAtomicUnit=on
  Chart1 : Stateflow chart  TreatAsAtomicUnit=on
  Logical Operator1 : Logic  Operator=NOT  AllPortsSameDT=off  OutDataTypeStr=boolean
  Logical Operator2 : Logic  Inputs=3  AllPortsSameDT=off  OutDataTypeStr=boolean
  Logical Operator3 : Logic  Operator=OR  AllPortsSameDT=off  OutDataTypeStr=boolean
  PA_KeSMSuSecRwStFtrstUpwdDnwdPosDelta_Val : Constant  Value=KeSMSuSecRwStFtrstUpwdDnwdPosDelta_Val
  PA_KeSMSuSecRwStLegrestInOutPosDelta_Val : Constant  Value=KeSMSuSecRwStLegrestInOutPosDelta_Val
  PA_KeSMSw4SSecRwLtStLgrstOtwdInwdClosePos1_Val : Constant  Value=KeSMSw4SSecRwLtStLgrstOtwdInwdClosePos1_Val
  PA_KeSMSw4SSecRwLtStLgrstUpwdDnwdClosePos1_Val : Constant  Value=KeSMSw4SSecRwLtStLgrstUpwdDnwdClosePos1_Val
  PA_KeSMSw4SSecRwLtStLgrstUpwdDnwdClosePos2_Val : Constant  Value=KeSMSw4SSecRwLtStLgrstUpwdDnwdClosePos2_Val
  R2Lt : Subsystem
  VIP_TrigJudg : Lib/VIP_TrigJudg  SystemSampleTime=-1
  R2Lt_TrgtPoss : Outport  VectorParamsAs1DForOutWhenUnconnected=on
  IfVeSMSuSecRwLtStRclCmdSrv_Val_writeRec : Outport  Port=2
  isAcsMdFeedBackNew_LyL : Outport  Port=3
  R2Lt_TrgtPoss_2 : Outport  Port=4  VectorParamsAs1DForOutWhenUnconnected=on
  wires:
  [failflg] -> Logical Operator3/2
  Logical Operator2/1 -> Logical Operator3/1
  [lgrstStep1_done] -> Logical Operator2/1
  [lgrstStep2_done] -> Logical Operator2/2
  [lgrstStep3_done] -> Logical Operator2/3
  Chart/4(failflg) -> [failflg]
  [KeSMSuSecRwStLegrestInOutPosDelta_Val] -> Chart/14(OtposDelta)
  PA_KeSMSuSecRwStLegrestInOutPosDelta_Val/1 -> [KeSMSuSecRwStLegrestInOutPosDelta_Val]
  Bus Selector5/3 -> [SecRwLtStHdrstFrwdBkwdPos]  "<IfVeSMSuSecRwLtStHdrstFrwdBkwdPos_Val_read>"
  isLfRecoveryArrivedAtTargetPos/1 -> Logical Operator1/1, [Recv_L_DoneOK]
  Logical Operator1/1 -> [Recv_L_DoneFailed]
  R2Lt/4(lgrstFtUpwd_ini) -> [lgrstStep3_ini]
  R2Lt/5(lgrstOtwd_ini) -> [lgrstStep1_ini]
  R2Lt/3(lgrstUpwd_ini) -> [lgrstStep2_ini]
  R2Lt/7(lgrstStep2_done) -> [lgrstStep3_done]
  R2Lt/8(lgrstStep3_done) -> [lgrstStep1_done]
  R2Lt/6(lgrstStep1_done) -> [lgrstStep2_done]
  [KeSMSuSecRwStFtrstUpwdDnwdPosDelta_Val] -> Chart/13(FtposDelta)
  PA_KeSMSuSecRwStFtrstUpwdDnwdPosDelta_Val/1 -> [KeSMSuSecRwStFtrstUpwdDnwdPosDelta_Val]
  [StepEn_LgrstStep2] -> R2Lt/9(StepEn_LgrstStep1)
  [StepEn_LgrstStep3] -> R2Lt/10(StepEn_LgrstStep2)
  [StepEn_LgrstStep1] -> R2Lt/11(StepEn_LgrstStep3)
  [SecRwLtStLgrstOtwdInwdPos] -> Chart/2(Otpos)
  [RrLtStFtUpwdDnwdPos] -> Chart/3(Ftpos)
  [CloseOtwdPos1] -> Chart/6(closeOtpos1)
  [CloseDnwdPos1] -> Chart/4(closedownpos1)
  [CloseDnwdPos2] -> Chart/5(closedownpos2)
  PA_KeSMSw4SSecRwLtStLgrstUpwdDnwdClosePos1_Val/1 -> [CloseDnwdPos1]
  PA_KeSMSw4SSecRwLtStLgrstUpwdDnwdClosePos2_Val/1 -> [CloseDnwdPos2]
  PA_KeSMSw4SSecRwLtStLgrstOtwdInwdClosePos1_Val/1 -> [CloseOtwdPos1]
  [lgrstStep3_done] -> Chart/9(Step3done)
  R2Lt/9(R2Lt_TrgtPoss_2) -> R2Lt_TrgtPoss_2/1
  Chart/3(StepEn_LgrstStep3) -> [StepEn_LgrstStep3]
  Chart/2(StepEn_LgrstStep2) -> [StepEn_LgrstStep2]
  Chart/1(StepEn_LgrstStep1) -> [StepEn_LgrstStep1]
  [lgrstStep2_done] -> Chart/8(Step2done)
  [lgrstStep3_ini] -> Chart/12(Step3_ini)
  [lgrstStep2_ini] -> Chart/11(Step2_ini)
  [lgrstStep1_ini] -> Chart/10(Step1_ini)
  [lgrstStep1_done] -> Chart/7(Step1done)
  [SecRwLtStLgrstUpwdDnwdPos] -> Chart/1(downpos)
  Bus Selector5/2 -> [RrLtStFtUpwdDnwdPos]  "<IfVeSMSuRrLtStFtUpwdDnwdPos_Val_read>"
  Bus Selector5/1 -> [SecRwLtStLgrstOtwdInwdPos]  "<IfVeSMSuSecRwLtStLgrstOtwdInwdPos_Val_read>"
  [PosV4s] -> Bus Selector6/1
  Bus Selector6/2 -> [RrLtStFtUpwdDnwdPosV]  "<IfVeSMSuRrLtStFtUpwdDnwdPosV_Val_read>"
  [Pos4s] -> Bus Selector5/1
  Bus Selector6/1 -> [SecRwLtStLgrstOtwdInwdPosV]  "<IfVeSMSuSecRwLtStLgrstOtwdInwdPosV_Val_read>"
  Bus Selector4/1 -> [SecRwLtStBkReclnUpwdDnwdPosV]  "<IfVeSMSuSecRwLtStBkReclnUpwdDnwdPosV_Val_read>"
  Bus Selector4/3 -> [SecRwLtStHPassStUpwdDnwdPosV]  "<IfVeSMSuSecRwLtStHPassStUpwdDnwdPosV_Val_read>"
  Bus Selector3/5 -> [SecRwLtStLtwdRtwdPos]  "<IfVeSMSuSecRwLtStLtwdRtwdPos_Val_read>"
  [Pos] -> Bus Selector3/1
  Bus Selector3/3 -> [SecRwLtStHPassStUpwdDnwdPos]  "<IfVeSMSuSecRwLtStHPassStUpwdDnwdPos_Val_read>"
  Bus Selector4/4 -> [SecRwLtStLgrstUpwdDnwdPosV]  "<IfVeSMSuSecRwLtStLgrstUpwdDnwdPosV_Val_read>"
  Bus Selector4/2 -> [SecRwLtStFrwdBkwdPosV]  "<IfVeSMSuSecRwLtStFrwdBkwdPosV_Val_read>"
  Bus Selector3/2 -> [SecRwLtStFrwdBkwdPos]  "<IfVeSMSuSecRwLtStFrwdBkwdPos_Val_read>"
  Bus Selector3/1 -> [SecRwLtStBkReclnUpwdDnwdPos]  "<IfVeSMSuSecRwLtStBkReclnUpwdDnwdPos_Val_read>"
  Bus Selector3/4 -> [SecRwLtStLgrstUpwdDnwdPos]  "<IfVeSMSuSecRwLtStLgrstUpwdDnwdPos_Val_read>"
  Bus Selector4/5 -> [SecRwLtStLtwdRtwdPosV]  "<IfVeSMSuSecRwLtStLtwdRtwdPosV_Val_read>"
  Bus Selector3/6 -> [R2LtStArmScrnPos]  "<IfVeSMSuSecRwLtStArmScrnPos_Val_read>"
  Bus Selector4/6 -> [R2LtStArmScrnPosV]  "<IfVeSMSuSecRwLtStArmScrnPosV_Val_read>"
  [PosV] -> Bus Selector4/1
  [SecRwLtStConfig4s] -> R2Lt/8(StConfig4s)
  Bus Selector2/2 -> [SecRwRtStConfig4s]  "<SecRwRtStConfig>"
  Bus Selector2/1 -> [SecRwLtStConfig4s]  "<SecRwLtStConfig>"
  StConfig4s/1 -> Bus Selector2/1
  SecRwLtStPossV4s/1 -> [PosV4s], R2Lt/7(SecRwLtStPossV4s)
  SecRwLtStsPoss4s/1 -> R2Lt/6(SecRwLtStsPoss4s), [Pos4s]
  Bus Selector/7 -> [ModeStCalib_2L4s]  "<Calib_2L4s>"
  Bus Selector/8 -> [ModeStCalib_2R4s]  "<Calib_2R4s>"
  [SecRwLtStConfig] -> R2Lt/5(StConfig)
  Bus Selector1/5 -> [ThdRwLtStConfig]  "<ThdRwLtStConfig>"
  Bus Selector1/2 -> [PassStConfig]  "<PassStConfig>"
  StConfig/1 -> Bus Selector1/1
  Bus Selector1/4 -> [SecRwRtStConfig]  "<SecRwRtStConfig>"
  Bus Selector1/3 -> [SecRwLtStConfig]  "<SecRwLtStConfig>"
  Bus Selector1/1 -> [DrvStConfig]  "<DrvStConfig>"
  Bus Selector1/6 -> [ThdRwRtStConfig]  "<ThdRwRtStConfig>"
  [Ly_L_DoneFailed] -> Bus Creator1/2  "isLgrstCloseLDoneFailed"
  [Ly_L_DoneOK] -> Bus Creator1/1  "isLgrstCloseLDoneOK"
  Bus Creator1/1 -> isAcsMdFeedBackNew_LyL/1
  [Recovery_Mod_Left] -> VIP_TrigJudg/1
  [ModeStCalib_2L4s] -> R2Lt/4(ModeStCalib_2L)
  ModeStCalib/1 -> Bus Selector/1
  Bus Selector/4 -> [ModeStCalib_2R]  "<Calib_2R>"
  Bus Selector/6 -> [ModeStCalib_3R]  "<Calib_3R>"
  Bus Selector/1 -> [ModeStCalib_Drv]  "<Calib_Drv>"
  Bus Selector/3 -> [ModeStCalib_2L]  "<Calib_2L>"
  Bus Selector/5 -> [ModeStCalib_3L]  "<Calib_3L>"
  Bus Selector/2 -> [ModeStCalib_Pass]  "<Calib_Pass>"
  Chart1/1(IfVeSMSuSecRwLtStRclCmdSrv_Val_write) -> IfVeSMSuSecRwLtStRclCmdSrv_Val_writeRec/1  "IfVeSMSuSecRwLtStRclCmdSrv_Val_write"
  Chart1/3(Md_L_DoneFailed) -> [Ly_L_DoneFailed]
  Chart1/2(Md_L_DoneOk) -> [Ly_L_DoneOK]
  [Recv_L_DoneFailed] -> Chart1/4(Md_L_DoneFailedRaw)
  [Recv_L_DoneOK] -> Chart1/3(Md_L_DoneOkRaw)
  SecRwLtStPossV/1 -> [PosV], R2Lt/3(SecRwLtStPossV)
  SecRwLtStsPoss/1 -> [Pos], R2Lt/2(SecRwLtStsPoss)
  R2Lt/1(R2Lt_TrgtPoss) -> R2Lt_TrgtPoss/1
  [EZE_TrigL] -> R2Lt/1(Mode_Trig)
  VIP_TrigJudg/1 -> [EZE_TrigL]
  Recovery_Mod_Left/1 -> [Recovery_Mod_Left]
  [IfVeSMSuSecRwLtStRclCmdSrv_Val_writeRaw] -> Chart1/2(IfVeSMSuSecRwLtStRclCmdSrv_Val_writeRaw)
  R2Lt/2(IfVeSMSuSecRwLtStRclCmdSrv_Val_writeRaw) -> [IfVeSMSuSecRwLtStRclCmdSrv_Val_writeRaw]
  Logical Operator3/1 -> Chart1/1(Left_Done)
